simulink model "MinigridBaseSimulationFile"  (R2024a)
settings: Solver=VariableStepAuto  StartTime=0.0  StopTime=T  RelTol=1e-3
PreLoadFcn:
  | % Qnom_bat = 26;
  | % eta_c = sqrt(0.9);
  | % eta_d = sqrt(0.9);
  | % A = 1;
  | % B = (100/Qnom_bat)*[eta_c -1/eta_d]*dt;
  | % C = 1;
  | % D = zeros(1,2);
  | % SOC_init = 10;
  | % Parameters = [A B C D eta_c eta_d SOC_init Qnom_bat];
  | % Batt.signals.values = Parameters;
  | % Batt.time = length(Parameters)';
  | % % t1 = 0.2 * [0:49]';
  | % % m = magic(10);
  | % % M = repmat(m,[1 1 length(t1)]);
  | % % data.time=t1;
  | % % data.signals.values = M;
  | % % data.signals.dimensions=[10 10];
  | % Batt.time = 1;
  | % v.Qnom_bat = 26;
  | % v.eta_c = sqrt(0.9);
  | % Batt.signals.values=v;
  | % % Batt.signals.values.eta_c = sqrt(0.9);
  | % % Batt.signals.values.eta_d = sqrt(0.9);
  | % % Batt.signals.values.A = 1;
  | % % Batt.signals.values.B = (100/Batt.signals.values.Qnom_bat)*[Batt.signals.values.eta_c -1/Batt.signals.values.eta_d]*dt;
  | % % Batt.signals.values.C = 1;
  | % % Batt.signals.values.D = zeros(1,2);
  | % % Batt.signals.values.SOC_init = 10;
undefined symbols (not defined in the file): Batt, Cp, Dair, dt, Electrolyzer, Grid, Tnom, Tstc, Ypv
libraries: spspowerguiLib x1
settings Model: Creator=USER  LastModifiedBy=USER

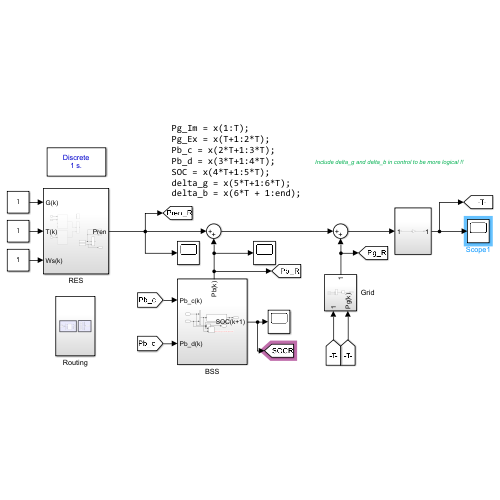
[thumbnail: Simulink's stored preview of the top-level diagram]
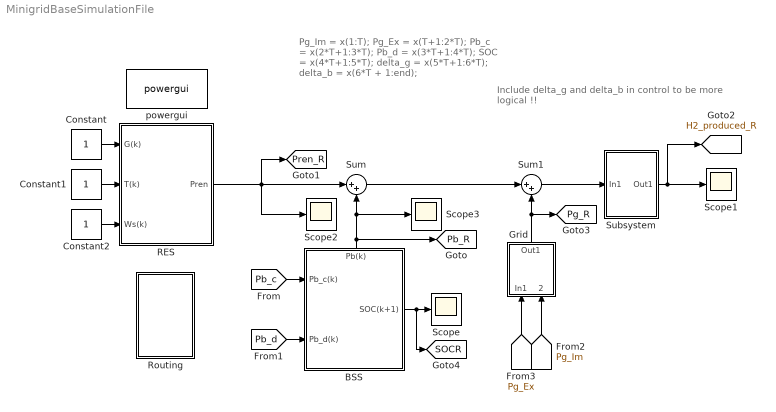
== system MinigridBaseSimulationFile ==
  note: Include delta_g and delta_b in control to be more logical !!
  note: Pg_Im = x(1:T);
      | Pg_Ex = x(T+1:2*T);
      | Pb_c = x(2*T+1:3*T);
      | Pb_d = x(3*T+1:4*T);
      | SOC = x(4*T+1:5*T);
      | delta_g = x(5*T+1:6*T);
      | delta_b = x(6*T + 1:end);
  BSS : Subsystem
      settings: PortSchema="{\"entries\":[{\"content\":{\"sides\":[{\"content\":{\"connectorIds\":[\"In1\",\"In2\"]},\"type\":\"ConnectorPlacement.EquallySpacedRectSide\",\"uuid\":\"4f2f7840-7969-468f-9b1c-20bf7095da3f\"},{\"content\":{\"connectorIds\":[\"Out1\"],\"side\":\"RIGHT\"},\"type\":\"ConnectorPlacement.EquallySpacedRectSide\",\"uuid\":\"5dca09d0-6cdb-46ae-891e-ce586056a4b2\"},{\"content\":{\"connectorIds\":[\"Out2\"],\"side\":\"TOP\"},\"type\":\"ConnectorPlacement.EquallySpacedRectSide\",\"uuid\":\"4e61ad00-dc85-42bf-b5e4-3229965ea073\"}]},\"type\":\"ConnectorPlacement.EquallySpacedConnector\",\"uuid\":\"822e1b7e-7a8b-4020-ad13-8f17d1212f4b\"}],\"packageUris\":[\"http://schema.mathworks.com/mf0/Connector/R2020b\"],\"version\":\"1.0\"}"
  Constant : Constant
  Constant1 : Constant
  Constant2 : Constant
  Grid : Subsystem
  RES : Subsystem
  Routing : Subsystem
  Scope{,1..3} (4 alike) : Scope
  Subsystem : Subsystem
  Sum : Sum  Inputs=|++
  Sum1 : Sum  Inputs=|++
  powergui : spspowerguiLib/powergui  Priority=1  SimulationMode=Discrete  SampleTime=dt  frequency=60  Iterations=50  frequencyindice=60  Pbase=100e6  ErrMax=1e-4  UnitsV=kV  UnitsW=MW  buscounter=0  FunctionMessages=off  echomessages=off  EnableUseOfTLC=off  CurrentSourceSwitches=off  DisableSnubberDevices=off  DisableRonSwitches=off  DisableVfSwitches=off  DisplayEquations=off  AutomaticDiscreteSolvers=off  SolverType=Tustin/Backward Euler (TBE)  Interpol=off  ExternalGateDelay=off  methode=off  Ts=100  x0status=blocks  SPID=on  SwTol=0  HookPort=off  NonlinearTolerance=1e-4  nMaxIteration=100  ContinueOnMaxIteration=off  RestoreLinks=warning  ResistiveCurrentMeasurement=off  Frange=[0:2:500]  Ylog=off  Xlog=on  ShowGrid=off  save=off  variable=ZData  structure=0  ZoomFFT=off  StartTime=0.0  cycles=1  DisplayStyle=1  fundamental=60  FreqAxis=off  MaxFrequency=1000  frequencyindicesteady=1  RmsSteady=1  display=off
  tag scope: H2_produced_R=global, Pb_R=global, Pg_R=global, Pren_R=global, SOCR=global
  wires:
  BSS/1(SOC(k+1)) -> [SOCR], Scope/1
  BSS/2(Pb(k)) -> Scope3/1, Sum/2, [Pb_R]
  RES/1(Pren) -> [Pren_R], Scope2/1, Sum/1
  Sum/1 -> Sum1/1
  Grid/1(Out1) -> [Pg_R], Sum1/2
  Sum1/1 -> Subsystem/1(In1)
  Constant/1 -> RES/1(G(k))
  Constant2/1 -> RES/3(Ws(k))
  Constant1/1 -> RES/2(T(k))
  Subsystem/1(Out1) -> [H2_produced_R], Scope1/1
  [Pg_Im] -> Grid/2(Pg(k))
  [Pb_c] -> BSS/1(Pb_c(k))
  [Pb_d] -> BSS/2(Pb_d(k))
  [Pg_Ex] -> Grid/1(In1)

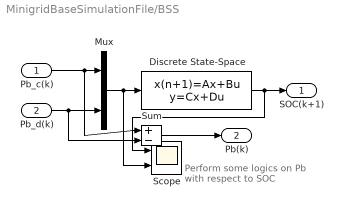
== system MinigridBaseSimulationFile/BSS ==
  note: Perform some logics on Pb with respect to SOC
  Pb_c(k) : Inport
  Pb_d(k) : Inport  Port=2
  Discrete State-Space : DiscreteStateSpace  A=Batt.signals.values(1)  B=Batt.signals.values(2:3)  C=Batt.signals.values(4)  D=Batt.signals.values(5:6)  InitialCondition=Batt.signals.values(7)  SampleTime=-1
  Mux : Mux  Inputs=2
  Scope : Scope  NumInputPorts=2
  Sum : Sum  Inputs=|+-
  SOC(k+1) : Outport
  Pb(k) : Outport  Port=2
  wires:
  Pb_c(k)/1 -> Sum/1, Mux/1
  Pb_d(k)/1 -> Sum/2, Mux/2
  Mux/1 -> Scope/2, Discrete State-Space/1
  Sum/1 -> Pb(k)/1
  Discrete State-Space/1 -> Scope/1, SOC(k+1)/1

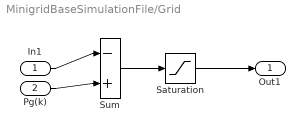
== system MinigridBaseSimulationFile/Grid ==
  In1 : Inport
  Pg(k) : Inport  Port=2
  Saturation : Saturate  UpperLimit=Grid.Pgrid_max  LowerLimit=Grid.Pgrid_min
  Sum : Sum  Inputs=|-+
  Out1 : Outport
  wires:
  Pg(k)/1 -> Sum/2
  Saturation/1 -> Out1/1
  In1/1 -> Sum/1
  Sum/1 -> Saturation/1

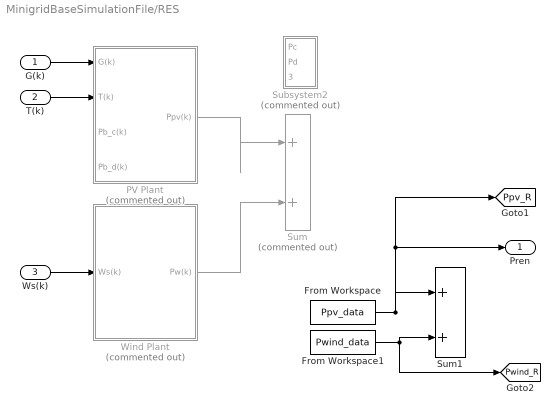
== system MinigridBaseSimulationFile/RES ==
  G(k) : Inport
  T(k) : Inport  Port=2
  Ws(k) : Inport  Port=3
  From Workspace : FromWorkspace  VariableName=Ppv_data  SampleTime=dt
  From Workspace1 : FromWorkspace  VariableName=Pwind_data  SampleTime=dt
  PV Plant : Subsystem  Commented=on
  Subsystem2 : Subsystem  Commented=on
  Sum : Sum  Commented=on  Inputs=|++
  Sum1 : Sum  Inputs=|++
  Wind Plant : Subsystem  Commented=on
  Pren : Outport
  tag scope: Ppv_R=global, Pwind_R=global
  wires:
  PV Plant/1(Ppv(k)) -> Sum/1
  G(k)/1 -> PV Plant/1(G(k))
  Ws(k)/1 -> Wind Plant/1(Ws(k))
  T(k)/1 -> PV Plant/2(T(k))
  Wind Plant/1(Pw(k)) -> Sum/2
  From Workspace1/1 -> [Pwind_R], Sum1/2
  From Workspace/1 -> [Ppv_R], Pren/1, Sum1/1

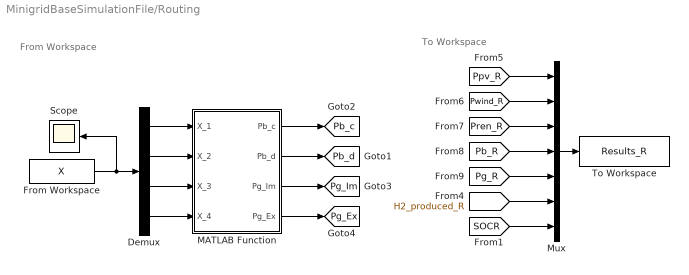
== system MinigridBaseSimulationFile/Routing ==
  note: From Workspace
  note: To Workspace
  Demux : Demux
  From Workspace : FromWorkspace  VariableName=X  SampleTime=dt
  MATLAB Function : MATLAB Function  TreatAsAtomicUnit=on
  Mux : Mux  Inputs=7
  Scope : Scope
  To Workspace : ToWorkspace  VariableName=Results_R  SampleTime=-1
  tag scope: Pb_c=global, Pb_d=global, Pg_Ex=global, Pg_Im=global
  wires:
  MATLAB Function/2(Pb_d) -> [Pb_d]
  MATLAB Function/4(Pg_Ex) -> [Pg_Ex]
  MATLAB Function/3(Pg_Im) -> [Pg_Im]
  MATLAB Function/1(Pb_c) -> [Pb_c]
  From Workspace/1 -> Demux/1, Scope/1
  Demux/1 -> MATLAB Function/1(X_1)
  Demux/2 -> MATLAB Function/2(X_2)
  Demux/3 -> MATLAB Function/3(X_3)
  Demux/4 -> MATLAB Function/4(X_4)
  [H2_produced_R] -> Mux/6
  [Pren_R] -> Mux/3
  [Pb_R] -> Mux/4
  [Ppv_R] -> Mux/1
  [Pg_R] -> Mux/5
  [Pwind_R] -> Mux/2
  Mux/1 -> To Workspace/1
  [SOCR] -> Mux/7

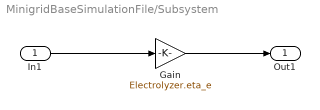
== system MinigridBaseSimulationFile/Subsystem ==
  In1 : Inport
  Gain : Gain  Gain=Electrolyzer.eta_e
  Out1 : Outport
  wires:
  In1/1 -> Gain/1
  Gain/1 -> Out1/1

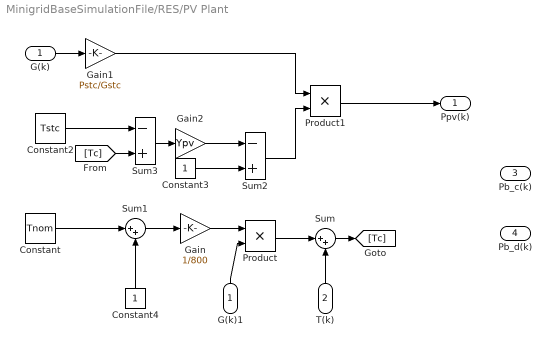
== system MinigridBaseSimulationFile/RES/PV Plant ==
  G(k) : Inport
  T(k) : Inport  Port=2
  Pb_c(k) : Inport  Port=3
  Pb_d(k) : Inport  Port=4
  Constant : Constant  Value=Tnom
  Constant2 : Constant  Value=Tstc
  Constant3 : Constant
  Constant4 : Constant
  G(k)1 : InportShadow
  Gain : Gain  Gain=1/800
  Gain1 : Gain  Gain=Pstc/Gstc
  Gain2 : Gain  Gain=Ypv
  Product : Product
  Product1 : Product
  Sum : Sum  Inputs=|++
  Sum1 : Sum  Inputs=|++
  Sum2 : Sum  Inputs=-+
  Sum3 : Sum  Inputs=-+
  Ppv(k) : Outport
  wires:
  Constant/1 -> Sum1/1
  Constant4/1 -> Sum1/2
  Sum1/1 -> Gain/1
  Gain/1 -> Product/1
  G(k)1/1 -> Product/2
  Product/1 -> Sum/1
  T(k)/1 -> Sum/2
  G(k)/1 -> Gain1/1
  Sum3/1 -> Gain2/1
  Gain2/1 -> Sum2/1
  Constant3/1 -> Sum2/2
  Product1/1 -> Ppv(k)/1
  Sum/1 -> [Tc]
  Constant2/1 -> Sum3/1
  [Tc] -> Sum3/2
  Sum2/1 -> Product1/2
  Gain1/1 -> Product1/1

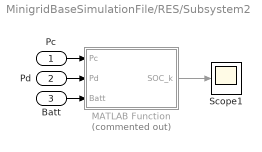
== system MinigridBaseSimulationFile/RES/Subsystem2 ==
  Pc : Inport
  Pd : Inport  Port=2
  Batt : Inport  Port=3
  MATLAB Function : MATLAB Function  Commented=on  TreatAsAtomicUnit=on
  Scope1 : Scope
  wires:
  MATLAB Function/1(SOC_k) -> Scope1/1
  Pd/1 -> MATLAB Function/2(Pd)
  Pc/1 -> MATLAB Function/1(Pc)
  Batt/1 -> MATLAB Function/3(Batt)

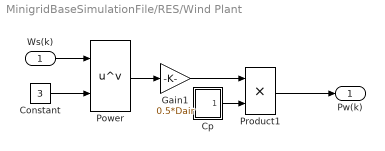
== system MinigridBaseSimulationFile/RES/Wind Plant ==
  Ws(k) : Inport
  Constant : Constant  Value=3
  Cp : Subsystem
  Gain1 : Gain  Gain=0.5*Dair
  Power : Math  Operator=pow
  Product1 : Product
  Pw(k) : Outport
  wires:
  Gain1/1 -> Product1/1
  Product1/1 -> Pw(k)/1
  Ws(k)/1 -> Power/1
  Power/1 -> Gain1/1
  Constant/1 -> Power/2
  Cp/1(Out1) -> Product1/2

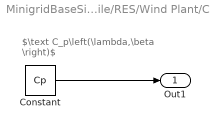
== system MinigridBaseSimulationFile/RES/Wind Plant/Cp ==
  note: $\text C_p\left(\lambda,\beta \right)$
  Constant : Constant  Value=Cp
  Out1 : Outport
  wires:
  Constant/1 -> Out1/1

== matlab function MinigridBaseSimulationFile/Routing/MATLAB Function ==
  data: X_1 input; Pb_c output; Pb_d output; Pg_Im output; Pg_Ex output; X_2 input; X_3 input; X_4 input
function [Pb_c, Pb_d, Pg_Im, Pg_Ex] = fcn(X_1, X_2, X_3, X_4)
    % x = X_.signals.values;
    Pg_Im = X_1; % X_1.signals.values(1);
    Pg_Ex = X_2; %X_2.signals.values(T+1);
    Pb_c = X_3; %X_3.signals.values(2*T+1);
    Pb_d = X_4; %X_4.signals.values(3*T+1);
    % SOC = x(4*T+1:5*T);
    % delta_g = x(5*T+1:6*T);
    % delta_b = x(6*T + 1:end);

== matlab function MinigridBaseSimulationFile/RES/Subsystem2/MATLAB Function ==
  data: Pc input; SOC_k output; Pd input; Batt input
function SOC_k = Battery(Pc, Pd, Batt)
persistent SOC_0

if isempty(SOC_0)
    SOC_0 = Batt.signals.values(7);
end

SOC_k = SOC_0 + (100/Batt.signals.values(10))*(Batt.signals.values(8)*Pc - Pd/Batt.signals.values(9))*dt;
